simulink model "flat_earth_6dof"  (R2020b)
settings: Solver=FixedStepAuto  StartTime=0.0  StopTime=400  FixedStep=1/1000  MaxStep=0.01  RelTol=1e-5
model workspace (MATLAB code in the model file + MAT data in the model file):
  aeroCoeff.Cl0 = 0.000591
  aeroCoeff.Cl_beta = -0.0618
  aeroCoeff.Cl_da = -0.09917
  aeroCoeff.Cl_da_alpha = -0.08269
  aeroCoeff.Cl_dr = 0.006934
  aeroCoeff.Cl_p = -0.5045
  aeroCoeff.Cl_r = 0.1695
  aeroCoeff.Cm0 = 0.09448
  aeroCoeff.Cm_alpha = -0.6028
  aeroCoeff.Cm_alpha2 = -2.14
  aeroCoeff.Cm_beta2 = 0.6921
  aeroCoeff.Cm_de = -1.921
  aeroCoeff.Cm_df = 0.4072
  aeroCoeff.Cm_q = -15.56
  aeroCoeff.Cm_r = -0.3118
  aeroCoeff.Cn0 = -0.003117
  aeroCoeff.Cn_beta = 0.006719
  aeroCoeff.Cn_beta3 = 0.1373
  aeroCoeff.Cn_da = -0.003872
  aeroCoeff.Cn_dr = -0.08265
  aeroCoeff.Cn_p = -0.1585
  aeroCoeff.Cn_q = 0.1595
  aeroCoeff.Cn_r = -0.1112
  aeroCoeff.Cx0 = -0.03554
  aeroCoeff.Cx_alpha = 0.00292
  aeroCoeff.Cx_alpha2 = 5.459
  aeroCoeff.Cx_alpha3 = -5.162
  aeroCoeff.Cx_df = -0.09447
  aeroCoeff.Cx_df_alpha = 1.106
  aeroCoeff.Cx_dr = 0.03412
  aeroCoeff.Cx_q = -0.6748
  aeroCoeff.Cy0 = -0.002226
  aeroCoeff.Cy_beta = -0.7678
  aeroCoeff.Cy_da = -0.02956
  aeroCoeff.Cy_dr = 0.1158
  aeroCoeff.Cy_dr_alpha = 0.5238
  aeroCoeff.Cy_p = -0.124
  aeroCoeff.Cy_r = 0.3666
  aeroCoeff.Cz0 = -0.05504
  aeroCoeff.Cz_alpha = -5.578
  aeroCoeff.Cz_alpha3 = 3.442
  aeroCoeff.Cz_de = -0.398
  aeroCoeff.Cz_de_beta = -15.93
  aeroCoeff.Cz_df = -1.377
  aeroCoeff.Cz_df_alpha = -1.261
  aeroCoeff.Cz_q = -2.988
  environment.EarthRefAlt = 0
  initCond.x0 = [0 0 0]
  initCond.v0 = [0 0 0]
  initCond.euler0 = [0 0 0]
  initCond.w0 = [0 0 0]
  inputs0.time = 0
  inputs0.signals(1).dimensions = 1
  inputs0.signals(1).values = 0
  inputs0.signals(2).dimensions = 1
  inputs0.signals(2).values = 0
  inputs0.signals(3).dimensions = 1
  inputs0.signals(3).values = 0
  states0.time = 0
  states0.signals(1).values = [0 0 -2202]
  states0.signals(1).dimensions = 3
  states0.signals(1).label = 'CSTATE'
  states0.signals(1).blockName = 'asb6DOFAirframeTemplate/6DOF EOM/6DOF (Euler Angles)/xe,ye,ze'
  states0.signals(1).stateName = ''
  states0.signals(1).inReferencedModel = 0
  states0.signals(1).sampleTime = [0 0]
  states0.signals(2).values = [0.128665353089 0.259337659946 -0.178947917154]
  states0.signals(2).dimensions = 3
  states0.signals(2).label = 'CSTATE'
  states0.signals(2).blockName = 'asb6DOFAirframeTemplate/6DOF EOM/6DOF (Euler Angles)/Calculate DCM &
    | Euler Angles/phi
    | theta
    | psi'
  states0.signals(2).stateName = ''
  states0.signals(2).inReferencedModel = 0
  states0.signals(2).sampleTime = [0 0]
  states0.signals(3).values = [36.9119692666 8.10720863264 8.82591882596]
  states0.signals(3).dimensions = 3
  states0.signals(3).label = 'CSTATE'
  states0.signals(3).blockName = 'asb6DOFAirframeTemplate/6DOF EOM/6DOF (Euler Angles)/ub,vb,wb'
  states0.signals(3).stateName = ''
  states0.signals(3).inReferencedModel = 0
  states0.signals(3).sampleTime = [0 0]
  states0.signals(4).values = [0 0 0]
  states0.signals(4).dimensions = 3
  states0.signals(4).label = 'CSTATE'
  states0.signals(4).blockName = 'asb6DOFAirframeTemplate/6DOF EOM/6DOF (Euler Angles)/p,q,r '
  states0.signals(4).stateName = ''
  states0.signals(4).inReferencedModel = 0
  states0.signals(4).sampleTime = [0 0]
  states0.signals(5).values = [0 0]
  states0.signals(5).dimensions = 2
  states0.signals(5).label = 'CSTATE'
  states0.signals(5).blockName = 'asb6DOFAirframeTemplate/Environment Model/Dryden Wind Turbulence Model 
    | (Continuous (+q +r))/Filters on velocities/Hwgw(s)/wg_p1'
  states0.signals(5).stateName = ''
  states0.signals(5).inReferencedModel = 0
  states0.signals(5).sampleTime = [0 0]
  states0.signals(6).values = [0 0]
  states0.signals(6).dimensions = 2
  states0.signals(6).label = 'CSTATE'
  states0.signals(6).blockName = 'asb6DOFAirframeTemplate/Environment Model/Dryden Wind Turbulence Model 
    | (Continuous (+q +r))/Filters on velocities/Hwgw(s)/wg_p2'
  states0.signals(6).stateName = ''
  states0.signals(6).inReferencedModel = 0
  states0.signals(6).sampleTime = [0 0]
  states0.signals(7).values = [0 0]
  states0.signals(7).dimensions = 2
  states0.signals(7).label = 'CSTATE'
  states0.signals(7).blockName = 'asb6DOFAirframeTemplate/Environment Model/Dryden Wind Turbulence Model 
    | (Continuous (+q +r))/Filters on velocities/Hvgw(s)/vg_p1'
  states0.signals(7).stateName = ''
  states0.signals(7).inReferencedModel = 0
  states0.signals(7).sampleTime = [0 0]
  states0.signals(8).values = [0 0]
  states0.signals(8).dimensions = 2
  states0.signals(8).label = 'CSTATE'
  states0.signals(8).blockName = 'asb6DOFAirframeTemplate/Environment Model/Dryden Wind Turbulence Model 
    | (Continuous (+q +r))/Filters on velocities/Hvgw(s)/vgw_p2'
  states0.signals(8).stateName = ''
  states0.signals(8).inReferencedModel = 0
  states0.signals(8).sampleTime = [0 0]
  states0.signals(9).values = [0 0]
  states0.signals(9).dimensions = 2
  states0.signals(9).label = 'CSTATE'
  states0.signals(9).blockName = 'asb6DOFAirframeTemplate/Environment Model/Dryden Wind Turbulence Model 
    | (Continuous (+q +r))/Filters on velocities/Hugw(s)/ug_p'
  states0.signals(9).stateName = ''
  states0.signals(9).inReferencedModel = 0
  states0.signals(9).sampleTime = [0 0]
  states0.signals(10).values = [0 0]
  states0.signals(10).dimensions = 2
  states0.signals(10).label = 'CSTATE'
  states0.signals(10).blockName = 'asb6DOFAirframeTemplate/Environment Model/Dryden Wind Turbulence Model 
    | (Continuous (+q +r))/Filters on angular rates/Hrgw/rgw_p'
  states0.signals(10).stateName = ''
  states0.signals(10).inReferencedModel = 0
  states0.signals(10).sampleTime = [0 0]
  states0.signals(11).values = [0 0]
  states0.signals(11).dimensions = 2
  states0.signals(11).label = 'CSTATE'
  states0.signals(11).blockName = 'asb6DOFAirframeTemplate/Environment Model/Dryden Wind Turbulence Model 
    | (Continuous (+q +r))/Filters on angular rates/Hqgw/qgw_p'
  states0.signals(11).stateName = ''
  states0.signals(11).inReferencedModel = 0
  states0.signals(11).sampleTime = [0 0]
  states0.signals(12).values = [0 0]
  states0.signals(12).dimensions = 2
  states0.signals(12).label = 'CSTATE'
  states0.signals(12).blockName = 'asb6DOFAirframeTemplate/Environment Model/Dryden Wind Turbulence Model 
    | (Continuous (+q +r))/Filters on angular rates/Hpgw/pgw_p'
  states0.signals(12).stateName = ''
  states0.signals(12).inReferencedModel = 0
  states0.signals(12).sampleTime = [0 0]
  vehicle.Sref = 23.23
  vehicle.cbar = 1.5875
  vehicle.bref = 14.63
  vehicle.CG = [0 0 0]
  vehicle.CP = [0 0 0]
  vehicle.inertia = [1  0  0; 0  0.144  0; 0  0  1]
  vehicle.acMass = 0.909090909091
  vehicle.Thrust = 2300
  vehicle.aileron_max = 0.523598775598
  vehicle.aileron_min = -0.523598775598
  vehicle.elevator_max = 0.523598775598
  vehicle.elevator_min = -0.523598775598
  vehicle.rudder_max = 1.0471975512
  vehicle.rudder_min = -1.0471975512
  other statements: initialize6DOFSkyHogg;
undefined symbols (not defined in the file or in its folder): Altitude_t, cgf, cgi, dref, mdot, mf, mi, sref, tburn, Thrusts
libraries: aerolibasang x6, aerolibatmos2 x2, shared6dof x1, aerolibwind2 x1
settings Model: SimulationMode=accelerator  Creator=natha  LastModifiedBy=natha
settings SolverCC: AutoInsertRateTranBlk=on  InsertRTBMode=Never (minimum delay)  MinimalZcImpactIntegration=on
settings DataIOCC: ExternalInput=inputs0  InitialState=states0  SaveFormat=Array  SaveOutput=off  ReturnWorkspaceOutputs=off
settings OptimizationCC: EnhancedBackFolding=on  StrengthReduction=on  InitFltsAndDblsToZero=on  DifferentSizesBufferReuse=on
settings DebuggingCC: WriteAfterWriteMsg=DisableAll  AlgebraicLoopMsg=none  FcnCallInpInsideContextMsg=warning  UnconnectedInputMsg=none  UnconnectedOutputMsg=none  UnconnectedLineMsg=none  UniqueDataStoreMsg=error  RootOutportRequireBusObject=none  StateNameClashWarn=warning  StrictBusMsg=ErrorOnBusTreatedAsVector  SFUnexpectedBacktrackingDiag=warning  SFNoUnconditionalDefaultTransitionDiag=warning  SFExecutionAtInitializationDiag=none  ArithmeticOperatorsInVariantConditions=warning
settings ModelReferenceCC: PropagateSignalLabelsOutOfModel=off
settings SFSimCC: SimUseLocalCustomCode=off
settings RTWCC: RTWUseLocalCustomCode=off
settings CodeAppCC: StateflowObjectComments=on

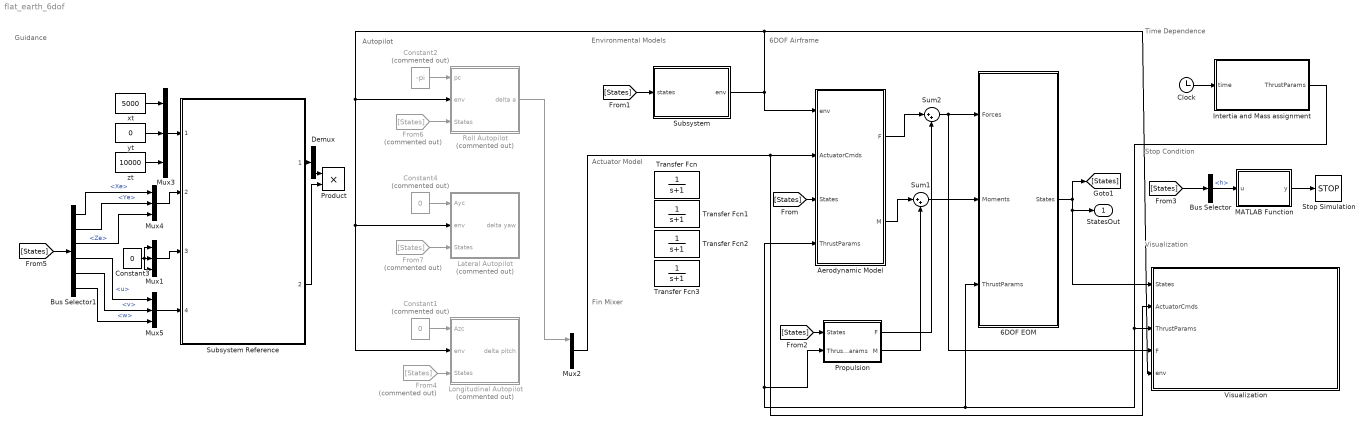
== system flat_earth_6dof ==
  note: 6DOF Airframe
  note: Environmental Models
  note: Autopilot
  note: Visualization
  note: Time Dependence
  note: Guidance
  note: Stop Condition
  note: Fin Mixer
  note: Actuator Model
  6DOF EOM : Subsystem  VariantControl=eom3DOF
  Aerodynamic Model : Subsystem  VariantControl=aeroCONST
  Bus Selector : BusSelector  OutputSignals=h
  Bus Selector1 : BusSelector  OutputSignals=Xe,Ye,Ze,u,v,w
  Clock : Clock
  Constant1 : Constant  Commented=on  Value=0
  Constant2 : Constant  Commented=on  Value=-pi
  Constant3 : Constant  Value=0
  Constant4 : Constant  Commented=on  Value=0
  Demux : Demux  Outputs=3
  From4 : From  Commented=on  GotoTag=States
  From6 : From  Commented=on  GotoTag=States
  From7 : From  Commented=on  GotoTag=States
  Intertia and Mass assignment : Subsystem
  Lateral Autopilot : Subsystem  Commented=on
  Longitudinal Autopilot : Subsystem  Commented=on
  MATLAB Function : MATLAB Function  TreatAsAtomicUnit=on
  Mux{1..5} (5 alike) : Mux  Inputs=3
  Product : Product
  Propulsion : Subsystem
      settings: RTWSystemCode=Inline
  Roll Autopilot : Subsystem  Commented=on
  Stop Simulation : Stop
  Subsystem : Subsystem
  Subsystem Reference : Subsystem  ReferencedSubsystem=PurePursuit
  Sum1 : Sum  Inputs=|++  InputSameDT=on  SaturateOnIntegerOverflow=on  OutDataTypeStr=Inherit: Same as first input
  Sum2 : Sum  Inputs=|++  InputSameDT=on  SaturateOnIntegerOverflow=on  OutDataTypeStr=Inherit: Same as first input
  Transfer Fcn{,1..3} (4 alike) : TransferFcn  Denominator=[1 1]
  Visualization : Subsystem
  xt : Constant  Value=5000
  yt : Constant  Value=0
  zt : Constant  Value=10000
  StatesOut : Outport  OutDataTypeStr=double  VectorParamsAs1DForOutWhenUnconnected=off
  wires:
  [States] -> Aerodynamic Model/3(States)
  Propulsion/2(M) -> Sum1/2
  [States] -> Propulsion/1(States)
  Intertia and Mass assignment/1(ThrustParams) -> 6DOF EOM/3(ThrustParams), Propulsion/2(ThrustParams), Aerodynamic Model/4(ThrustParams), Visualization/3(ThrustParams)
  Sum2/1 -> 6DOF EOM/1(Forces), Visualization/4(F)
  Aerodynamic Model/2(M) -> Sum1/1
  Propulsion/1(F) -> Sum2/2
  [States] -> Subsystem/1(states)
  Subsystem/1(env) -> Aerodynamic Model/1(env), Roll Autopilot/2(env), Lateral Autopilot/2(env), Longitudinal Autopilot/2(env), Visualization/5(env)
  MATLAB Function/1(y) -> Stop Simulation/1
  [States] -> Bus Selector/1
  Bus Selector/1 -> MATLAB Function/1(u)  "<h>"
  Clock/1 -> Intertia and Mass assignment/1(time)
  From4/1 -> Longitudinal Autopilot/3(States)
  Aerodynamic Model/1(F) -> Sum2/1
  Sum1/1 -> 6DOF EOM/2(Moments)
  Mux1/1 -> Subsystem Reference/3
  Constant3/1 -> Mux1/1, Mux1/2, Mux1/3
  Mux3/1 -> Subsystem Reference/1
  zt/1 -> Mux3/3
  yt/1 -> Mux3/2
  xt/1 -> Mux3/1
  [States] -> Bus Selector1/1
  Mux4/1 -> Subsystem Reference/2
  Bus Selector1/1 -> Mux4/1  "<Xe>"
  Bus Selector1/2 -> Mux4/2  "<Ye>"
  Bus Selector1/3 -> Mux4/3  "<Ze>"
  Mux5/1 -> Subsystem Reference/4
  Bus Selector1/4 -> Mux5/1  "<u>"
  Bus Selector1/5 -> Mux5/2  "<v>"
  Bus Selector1/6 -> Mux5/3  "<w>"
  Subsystem Reference/1 -> Demux/1
  Subsystem Reference/2 -> Product/2
  Demux/3 -> Product/1
  6DOF EOM/1(States) -> Visualization/1(States), StatesOut/1, [States]
  Constant1/1 -> Longitudinal Autopilot/1(Azc)
  Mux2/1 -> Aerodynamic Model/2(ActuatorCmds), Visualization/2(ActuatorCmds)
  From6/1 -> Roll Autopilot/3(States)
  From7/1 -> Lateral Autopilot/3(States)
  Constant4/1 -> Lateral Autopilot/1(Ayc)
  Constant2/1 -> Roll Autopilot/1(pc)
  Roll Autopilot/1(delta a) -> Mux2/1

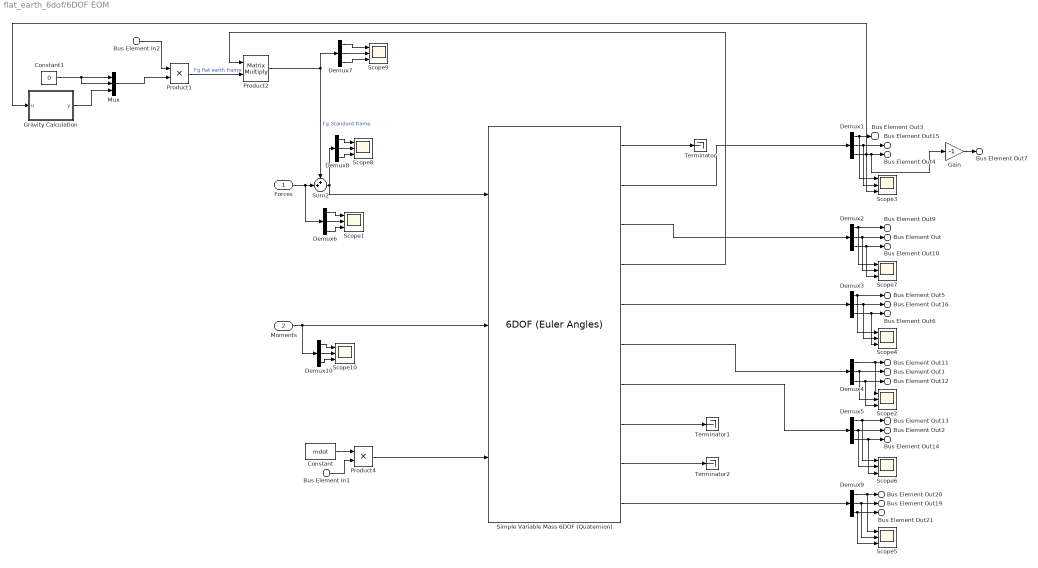
== system flat_earth_6dof/6DOF EOM ==
  Forces : Inport
  Moments : Inport  Port=2
  Bus Element In2 : Inport  Port=3  PortName=ThrustParams  Element=mass
  Bus Element In1 : Inport  Port=3  PortName=ThrustParams  Element=ThrustOn
  Constant : Constant  Value=mdot
  Constant1 : Constant  Value=0
  Demux{1..10} (10 alike) : Demux  Outputs=3
  Gain : Gain  Gain=-1
  Gravity Calculation : MATLAB Function  TreatAsAtomicUnit=on
  Mux : Mux  Inputs=3
  Product1 : Product
  Product2 : Product  Multiplication=Matrix(*)
  Product4 : Product
  Scope{1..10} (10 alike) : Scope  NumInputPorts=3
  Simple Variable Mass 6DOF (Quaternion) : shared6dof/6DOF (Euler Angles)  units=Metric (MKS)  mtype=Simple Variable  rep=Quaternion  xme_0=[0 0 -10000]  Vm_0=[0.0001 0 0]  eul_0=[0 45*(pi/180) 0]  pm_0=[0 0 0]  mass_0=mi  mass_e=mf  mass_f=mi  inertia=eye(3)  inertia_e=If  inertia_f=Ii  k_quat=1.0  vre_flag=off  abi_flag=on  aMode=0  xme_statename=''  Vm_statename=''  eul_statename=''  quat_statename=''  pm_statename=''  mass_statename=''
      settings: SourceProductBaseCode=AE,PW,MT,UV,VE,VP
  Sum2 : Sum  Inputs=++|  InputSameDT=on  SaturateOnIntegerOverflow=on  OutDataTypeStr=Inherit: Same as first input
  Terminator : Terminator
  Terminator1 : Terminator
  Terminator2 : Terminator
  Bus Element Out3 : Outport  VectorParamsAs1DForOutWhenUnconnected=off  PortName=States  Element=Xe
  Bus Element Out4 : Outport  VectorParamsAs1DForOutWhenUnconnected=off  PortName=States  Element=Ze
  Bus Element Out : Outport  VectorParamsAs1DForOutWhenUnconnected=off  PortName=States  Element=theta
  Bus Element Out5 : Outport  VectorParamsAs1DForOutWhenUnconnected=off  PortName=States  Element=u
  Bus Element Out6 : Outport  VectorParamsAs1DForOutWhenUnconnected=off  PortName=States  Element=w
  Bus Element Out1 : Outport  VectorParamsAs1DForOutWhenUnconnected=off  PortName=States  Element=q
  Bus Element Out2 : Outport  VectorParamsAs1DForOutWhenUnconnected=off  PortName=States  Element=q_dot
  Bus Element Out15 : Outport  VectorParamsAs1DForOutWhenUnconnected=off  PortName=States  Element=Ye
  Bus Element Out9 : Outport  VectorParamsAs1DForOutWhenUnconnected=off  PortName=States  Element=phi
  Bus Element Out10 : Outport  VectorParamsAs1DForOutWhenUnconnected=off  PortName=States  Element=psi
  Bus Element Out16 : Outport  VectorParamsAs1DForOutWhenUnconnected=off  PortName=States  Element=v
  Bus Element Out11 : Outport  VectorParamsAs1DForOutWhenUnconnected=off  PortName=States  Element=p
  Bus Element Out12 : Outport  VectorParamsAs1DForOutWhenUnconnected=off  PortName=States  Element=r
  Bus Element Out13 : Outport  VectorParamsAs1DForOutWhenUnconnected=off  PortName=States  Element=p_dot
  Bus Element Out14 : Outport  VectorParamsAs1DForOutWhenUnconnected=off  PortName=States  Element=r_dot
  Bus Element Out19 : Outport  VectorParamsAs1DForOutWhenUnconnected=off  PortName=States  Element=Ay
  Bus Element Out20 : Outport  VectorParamsAs1DForOutWhenUnconnected=off  PortName=States  Element=Ax
  Bus Element Out21 : Outport  VectorParamsAs1DForOutWhenUnconnected=off  PortName=States  Element=Az
  Bus Element Out7 : Outport  VectorParamsAs1DForOutWhenUnconnected=off  PortName=States  Element=h
  wires:
  Demux5/3 -> Scope6/3, Bus Element Out14/1
  Demux5/2 -> Bus Element Out2/1, Scope6/2
  Demux4/3 -> Scope2/3, Bus Element Out12/1
  Demux4/2 -> Bus Element Out1/1, Scope2/2
  Demux4/1 -> Scope2/1, Bus Element Out11/1
  Demux3/3 -> Scope4/3, Bus Element Out6/1
  Demux3/2 -> Scope4/2, Bus Element Out16/1
  Demux3/1 -> Scope4/1, Bus Element Out5/1
  Demux2/3 -> Scope7/3, Bus Element Out10/1
  Demux2/2 -> Scope7/2, Bus Element Out/1
  Demux2/1 -> Bus Element Out9/1, Scope7/1
  Demux1/3 -> Gravity Calculation/1(u), Scope3/3, Gain/1, Bus Element Out4/1
  Demux1/2 -> Scope3/2, Bus Element Out15/1
  Moments/1 -> Demux10/1, Simple Variable Mass 6DOF (Quaternion)/2
  Forces/1 -> Demux6/1, Sum2/2
  Bus Element In2/1 -> Product1/1
  Demux1/1 -> Scope3/1, Bus Element Out3/1
  Sum2/1 -> Simple Variable Mass 6DOF (Quaternion)/1, Demux8/1
  Demux9/2 -> Scope5/2, Bus Element Out19/1
  Demux9/3 -> Bus Element Out21/1, Scope5/3
  Demux9/1 -> Scope5/1, Bus Element Out20/1
  Demux5/1 -> Scope6/1, Bus Element Out13/1
  Demux6/1 -> Scope1/1
  Demux6/3 -> Scope1/3
  Demux6/2 -> Scope1/2
  Demux8/3 -> Scope8/3
  Demux8/2 -> Scope8/2
  Demux8/1 -> Scope8/1
  Demux10/1 -> Scope10/1
  Demux10/2 -> Scope10/2
  Demux10/3 -> Scope10/3
  Demux7/2 -> Scope9/2
  Demux7/3 -> Scope9/3
  Demux7/1 -> Scope9/1
  Product2/1 -> Demux7/1, Sum2/1  "Fg Standard frame"
  Bus Element In1/1 -> Product4/2
  Constant/1 -> Product4/1
  Product4/1 -> Simple Variable Mass 6DOF (Quaternion)/3
  Constant1/1 -> Mux/2, Mux/1
  Product1/1 -> Product2/2  "Fg flat earth frame"
  Mux/1 -> Product1/2
  Gravity Calculation/1(y) -> Mux/3
  Simple Variable Mass 6DOF (Quaternion)/1 -> Terminator/1
  Simple Variable Mass 6DOF (Quaternion)/2 -> Demux1/1
  Simple Variable Mass 6DOF (Quaternion)/3 -> Demux2/1
  Simple Variable Mass 6DOF (Quaternion)/4 -> Product2/1
  Simple Variable Mass 6DOF (Quaternion)/5 -> Demux3/1
  Simple Variable Mass 6DOF (Quaternion)/6 -> Demux4/1
  Simple Variable Mass 6DOF (Quaternion)/7 -> Demux5/1
  Simple Variable Mass 6DOF (Quaternion)/9 -> Terminator2/1
  Simple Variable Mass 6DOF (Quaternion)/8 -> Terminator1/1
  Simple Variable Mass 6DOF (Quaternion)/10 -> Demux9/1
  Gain/1 -> Bus Element Out7/1

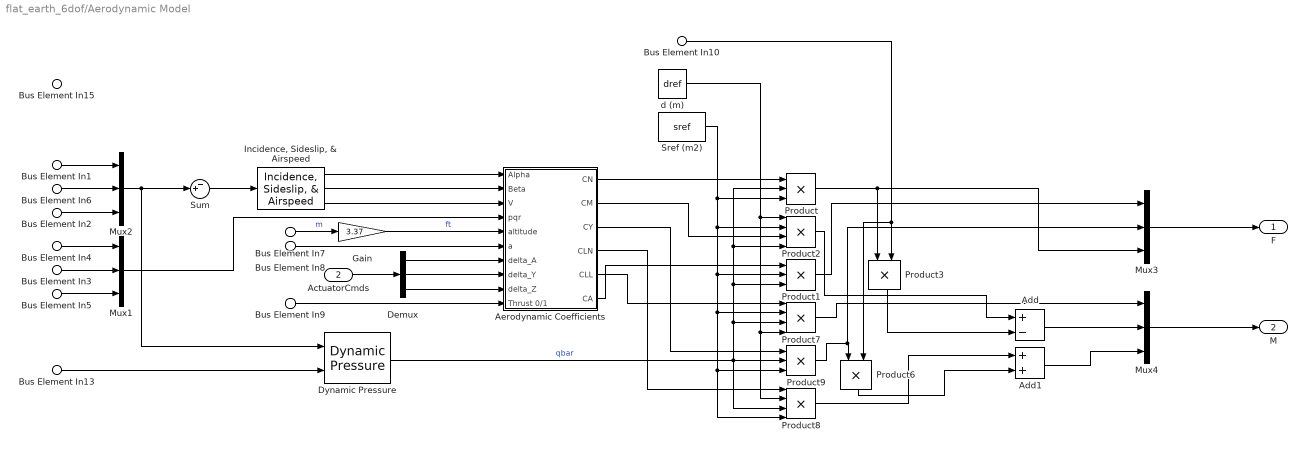
== system flat_earth_6dof/Aerodynamic Model ==
  Bus Element In13 : Inport  PortName=env  Element=rho
  Bus Element In8 : Inport  PortName=env  Element=a
  Bus Element In15 : Inport  PortName=env  Element=Vwind
  ActuatorCmds : Inport  Port=2
  Bus Element In1 : Inport  Port=3  PortName=States  Element=u
  Bus Element In2 : Inport  Port=3  PortName=States  Element=w
  Bus Element In3 : Inport  Port=3  PortName=States  Element=q
  Bus Element In6 : Inport  Port=3  PortName=States  Element=v
  Bus Element In4 : Inport  Port=3  PortName=States  Element=p
  Bus Element In5 : Inport  Port=3  PortName=States  Element=r
  Bus Element In7 : Inport  Port=3  PortName=States  Element=h
  Bus Element In9 : Inport  Port=4  PortName=ThrustParams  Element=ThrustOn
  Bus Element In10 : Inport  Port=4  PortName=ThrustParams  Element=cg
  Add : Sum  Inputs=+-
  Add1 : Sum
  Aerodynamic Coefficients : Subsystem
  Demux : Demux  Outputs=3
  Dynamic Pressure : aerolibasang/Dynamic Pressure
  Gain : Gain  Gain=3.37
  "Incidence, Sideslip, & Airspeed" : aerolibasang/Incidence, Sideslip, & Airspeed
  Mux{1..4} (4 alike) : Mux  Inputs=3
  Product : Product  Inputs=3
  Product1 : Product  Inputs=3
  Product2 : Product  Inputs=4
  Product3 : Product
  Product6 : Product
  Product7 : Product  Inputs=4
  Product8 : Product  Inputs=4
  Product9 : Product  Inputs=3
  Sref (m2) : Constant  Value=sref
  Sum : Sum  Inputs=-+|
  d (m) : Constant  Value=dref
  F : Outport  Unit=N  VectorParamsAs1DForOutWhenUnconnected=off
  M : Outport  Port=2  Unit=N*m  VectorParamsAs1DForOutWhenUnconnected=off
  wires:
  Bus Element In5/1 -> Mux1/3
  Bus Element In3/1 -> Mux1/2
  Bus Element In4/1 -> Mux1/1
  Mux1/1 -> Aerodynamic Coefficients/4(pqr)
  Mux2/1 -> Sum/2, Dynamic Pressure/1
  Dynamic Pressure/1 -> Product7/3, Product1/3, Product2/4, Product/2, Product8/3, Product9/2  "qbar"
  Bus Element In13/1 -> Dynamic Pressure/2
  "Incidence, Sideslip, & Airspeed"/3 -> Aerodynamic Coefficients/3(V)
  Bus Element In1/1 -> Mux2/1
  Bus Element In6/1 -> Mux2/2
  Bus Element In2/1 -> Mux2/3
  ActuatorCmds/1 -> Demux/1
  Demux/2 -> Aerodynamic Coefficients/8(delta_Y)
  Bus Element In8/1 -> Aerodynamic Coefficients/6(a)
  Sref (m2)/1 -> Product/3, Product8/4, Product9/3, Product7/2, Product1/2, Product2/2
  d (m)/1 -> Product8/2, Product7/4, Product2/1
  Product2/1 -> Add/1
  Product3/1 -> Add/2
  Bus Element In10/1 -> Product6/2, Product3/2
  Product1/1 -> Mux3/1
  Bus Element In7/1 -> Gain/1  "m"
  "Incidence, Sideslip, & Airspeed"/1 -> Aerodynamic Coefficients/1(Alpha)
  Product/1 -> Mux3/3, Product3/1
  Mux3/1 -> F/1
  Mux4/1 -> M/1
  "Incidence, Sideslip, & Airspeed"/2 -> Aerodynamic Coefficients/2(Beta)
  Aerodynamic Coefficients/1(CN) -> Product/1
  Aerodynamic Coefficients/2(CM) -> Product2/3
  Aerodynamic Coefficients/6(CA) -> Product1/1
  Product6/1 -> Add1/2
  Aerodynamic Coefficients/5(CLL) -> Product7/1
  Product7/1 -> Mux4/1
  Add1/1 -> Mux4/3
  Product9/1 -> Mux3/2, Product6/1
  Add/1 -> Mux4/2
  Product8/1 -> Add1/1
  Demux/3 -> Aerodynamic Coefficients/9(delta_Z)
  Gain/1 -> Aerodynamic Coefficients/5(altitude)  "ft"
  Sum/1 -> "Incidence, Sideslip, & Airspeed"/1
  Bus Element In9/1 -> Aerodynamic Coefficients/10(Thrust 0/1)
  Demux/1 -> Aerodynamic Coefficients/7(delta_A)
  Aerodynamic Coefficients/4(CLN) -> Product8/1
  Aerodynamic Coefficients/3(CY) -> Product9/1

== system flat_earth_6dof/Intertia and Mass assignment ==
  time : Inport
  Constant : Constant  Value=tburn
  Constant1 : Constant  Value=mi
  Constant2 : Constant  Value=mf
  Constant3 : Constant  Value=mdot
  Constant4 : Constant  Value=cgi
  Constant5 : Constant  Value=cgf
  MATLAB Function1 : MATLAB Function  TreatAsAtomicUnit=on
  MATLAB Function2 : MATLAB Function  TreatAsAtomicUnit=on
  MATLAB Function3 : MATLAB Function  TreatAsAtomicUnit=on
  Mux : Mux  Inputs=7
  Out Bus Element : Outport  PortName=ThrustParams  Element=ThrustOn
  Out Bus Element1 : Outport  PortName=ThrustParams  Element=mass
  Out Bus Element2 : Outport  PortName=ThrustParams  Element=cg
  wires:
  MATLAB Function2/1(y) -> Out Bus Element/1
  MATLAB Function1/1(y) -> Out Bus Element1/1
  MATLAB Function3/1(y) -> Out Bus Element2/1
  Constant2/1 -> Mux/4
  Constant1/1 -> Mux/3
  Constant/1 -> Mux/2
  time/1 -> Mux/1
  Constant3/1 -> Mux/5
  Constant4/1 -> Mux/6
  Constant5/1 -> Mux/7
  Mux/1 -> MATLAB Function3/1(u), MATLAB Function2/1(u), MATLAB Function1/1(u)

== system flat_earth_6dof/Lateral Autopilot ==
  Ayc : Inport
  env : Inport  Port=2
  States : Inport  Port=3
  3 loop autopilot : Subsystem
  Gain Scheduler : Subsystem
  delta yaw : Outport
  wires:
  Gain Scheduler/4(kss) -> 3 loop autopilot/6(kss)
  3 loop autopilot/1(delta yaw) -> delta yaw/1
  env/1 -> Gain Scheduler/1(env)
  Ayc/1 -> 3 loop autopilot/2(Ayc)
  Gain Scheduler/1(k1) -> 3 loop autopilot/3(k1)
  Gain Scheduler/3(k3) -> 3 loop autopilot/5(k3)
  Gain Scheduler/2(k2) -> 3 loop autopilot/4(k2)
  States/1 -> Gain Scheduler/2(States), 3 loop autopilot/1(States)

== system flat_earth_6dof/Longitudinal Autopilot ==
  Azc : Inport
  env : Inport  Port=2
  States : Inport  Port=3
  3 loop autopilot : Subsystem
  Gain Scheduler : Subsystem
  Scope : Scope
  delta pitch : Outport
  wires:
  Gain Scheduler/4(kss) -> 3 loop autopilot/6(kss)
  3 loop autopilot/1(deltap) -> Scope/1, delta pitch/1  "Pitch"
  env/1 -> Gain Scheduler/1(env)
  States/1 -> Gain Scheduler/2(States), 3 loop autopilot/1(States)
  Azc/1 -> 3 loop autopilot/2(Azc)
  Gain Scheduler/1(k1) -> 3 loop autopilot/3(k1)
  Gain Scheduler/3(k3) -> 3 loop autopilot/5(k3)
  Gain Scheduler/2(k2) -> 3 loop autopilot/4(k2)

== system flat_earth_6dof/Propulsion ==
  Bus Element In : Inport  PortName=States  Element=h
  Bus Element In2 : Inport  Port=2  PortName=ThrustParams  Element=ThrustOn
  Constant : Constant  Value=0
  Constant1 : Constant  Value=0
  Mux : Mux  Inputs=3
  Product : Product
  ThrustX : Lookup_n-D  NumberOfTableDimensions=1  LookupTableObject=''  BreakpointsForDimension1=Altitude_t  IndexSearchMethod=Linear search  BeginIndexSearchUsingPreviousIndexResult=on  Table=Thrusts  ExtrapMethod=Clip  UseLastTableValue=on  InputSameDT=on
  Thrust_M1 : Constant  Value=[0 0 0]'  SampleTime=-1
  F : Outport  Unit=N  VectorParamsAs1DForOutWhenUnconnected=off
  M : Outport  Port=2  Unit=N*m  VectorParamsAs1DForOutWhenUnconnected=off
  wires:
  Thrust_M1/1 -> M/1
  Mux/1 -> F/1
  ThrustX/1 -> Product/1
  Bus Element In2/1 -> Product/2
  Product/1 -> Mux/1
  Constant1/1 -> Mux/3
  Constant/1 -> Mux/2
  Bus Element In/1 -> ThrustX/1

== system flat_earth_6dof/Roll Autopilot ==
  pc : Inport
  env : Inport  Port=2
  States : Inport  Port=3
  Gain Scheduler : Subsystem
  Roll autopilot : Subsystem
  delta a : Outport
  wires:
  Roll autopilot/1(delta a) -> delta a/1  "delta a"
  env/1 -> Gain Scheduler/1(env)
  States/1 -> Roll autopilot/1(States), Gain Scheduler/2(States)
  pc/1 -> Roll autopilot/2(pc)
  Gain Scheduler/1(k1) -> Roll autopilot/3(k1)
  Gain Scheduler/2(k2) -> Roll autopilot/4(k2)
  Gain Scheduler/3(kss) -> Roll autopilot/5(kss)

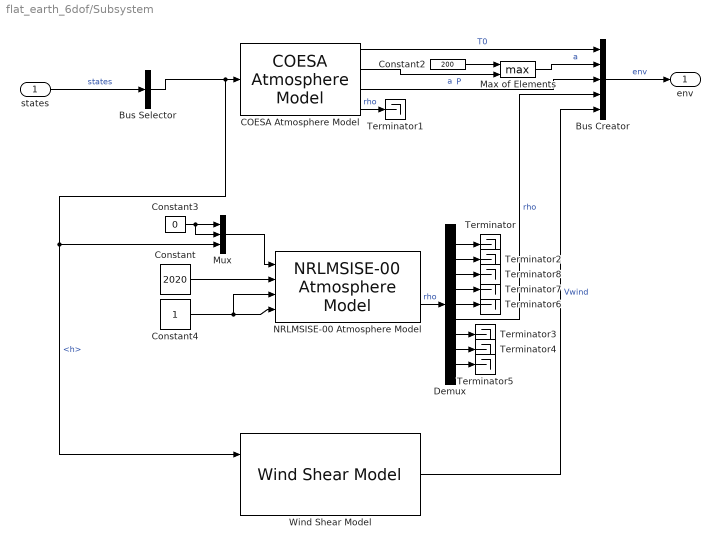
== system flat_earth_6dof/Subsystem ==
  states : Inport
  Bus Creator : BusCreator  Inputs=5
  Bus Selector : BusSelector  OutputSignals=h
  COESA Atmosphere Model : aerolibatmos2/COESA Atmosphere Model  units=Metric (MKS)  spec=1976 COESA-extended U.S. Standard Atmosphere  model=Profile  profile_var=High temperature  profile_percent=1%  profile_alt=5 km (16404 ft)  envelope_var=High temperature  envelope_percent=1%  action=Warning
  Constant : Constant  Value=2020
  Constant2 : Constant  Value=200
  Constant3 : Constant  Value=0
  Constant4 : Constant
  Demux : Demux  Outputs=9
  Max of Elements : MinMax  Function=max  Inputs=2
  Mux : Mux  Inputs=3
  NRLMSISE-00 Atmosphere Model : aerolibatmos2/NRLMSISE-00 Atmosphere Model  units=Metric (MKS)  lst_input=off  flux_ap_input=off  flags_input=Internal  flags=ones(1,23)  oxygen_in=off  action=Warning
      settings: SourceProductBaseCode=AE
  Terminator{,1..8} (9 alike) : Terminator
  Wind Shear Model : aerolibwind2/Wind Shear Model  units=Metric (MKS)  phase=Category C - Terminal Flight Phase  W_20=15  Wdeg=0
  env : Outport
  wires:
  states/1 -> Bus Selector/1  "states"
  COESA Atmosphere Model/3 -> Bus Creator/3  "P"
  COESA Atmosphere Model/2 -> Max of Elements/2  "a"
  Bus Selector/1 -> COESA Atmosphere Model/1, Mux/3, Wind Shear Model/1  "<h>"
  Bus Creator/1 -> env/1  "env"
  COESA Atmosphere Model/1 -> Bus Creator/1  "T0"
  Max of Elements/1 -> Bus Creator/2  "a"
  Constant2/1 -> Max of Elements/1
  Mux/1 -> NRLMSISE-00 Atmosphere Model/1
  Constant3/1 -> Mux/2, Mux/1
  Constant/1 -> NRLMSISE-00 Atmosphere Model/2
  Constant4/1 -> NRLMSISE-00 Atmosphere Model/3, NRLMSISE-00 Atmosphere Model/4
  NRLMSISE-00 Atmosphere Model/2 -> Demux/1  "rho"
  Demux/6 -> Bus Creator/4  "rho"
  Demux/1 -> Terminator/1
  COESA Atmosphere Model/4 -> Terminator1/1  "rho"
  Demux/2 -> Terminator2/1
  Demux/3 -> Terminator8/1
  Demux/4 -> Terminator7/1
  Demux/5 -> Terminator6/1
  Demux/7 -> Terminator3/1
  Demux/8 -> Terminator4/1
  Demux/9 -> Terminator5/1
  Wind Shear Model/1 -> Bus Creator/5  "Vwind"

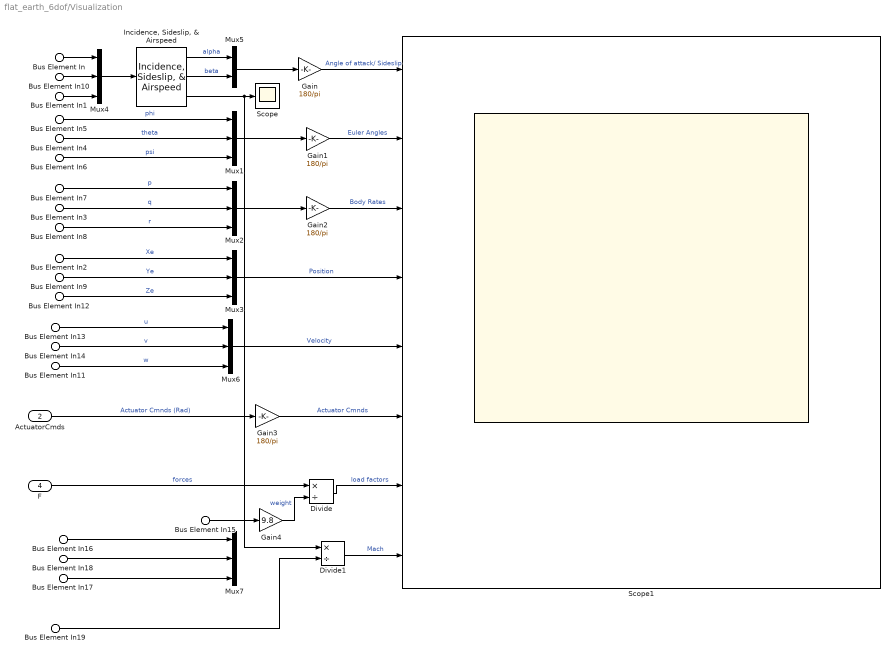
== system flat_earth_6dof/Visualization ==
  Bus Element In : Inport  PortName=States  Element=u
  Bus Element In13 : Inport  PortName=States  Element=u
  Bus Element In1 : Inport  PortName=States  Element=w
  Bus Element In11 : Inport  PortName=States  Element=w
  Bus Element In3 : Inport  PortName=States  Element=q
  Bus Element In4 : Inport  PortName=States  Element=theta
  Bus Element In12 : Inport  PortName=States  Element=Ze
  Bus Element In2 : Inport  PortName=States  Element=Xe
  Bus Element In10 : Inport  PortName=States  Element=v
  Bus Element In14 : Inport  PortName=States  Element=v
  Bus Element In5 : Inport  PortName=States  Element=phi
  Bus Element In6 : Inport  PortName=States  Element=psi
  Bus Element In7 : Inport  PortName=States  Element=p
  Bus Element In8 : Inport  PortName=States  Element=r
  Bus Element In9 : Inport  PortName=States  Element=Ye
  Bus Element In16 : Inport  PortName=States  Element=Ax
  Bus Element In18 : Inport  PortName=States  Element=Ay
  Bus Element In17 : Inport  PortName=States  Element=Az
  ActuatorCmds : Inport  Port=2
  Bus Element In15 : Inport  Port=3  PortName=ThrustParams  Element=mass
  F : Inport  Port=4
  Bus Element In19 : Inport  Port=5  PortName=env  Element=a
  Divide : Product  Inputs=*/
  Divide1 : Product  Inputs=*/
  Gain{,1..3} (4 alike) : Gain  Gain=180/pi
  Gain4 : Gain  Gain=9.8
  "Incidence, Sideslip, & Airspeed" : aerolibasang/Incidence, Sideslip, & Airspeed
  Mux{1..4,6..7} (6 alike) : Mux  Inputs=3
  Mux5 : Mux  Inputs=2
  Scope : Scope
  Scope1 : Scope  NumInputPorts=8
  wires:
  Mux3/1 -> Scope1/4  "Position"
  Bus Element In2/1 -> Mux3/1  "Xe"
  Bus Element In9/1 -> Mux3/2  "Ye"
  Bus Element In12/1 -> Mux3/3  "Ze"
  Mux2/1 -> Gain2/1
  Mux1/1 -> Gain1/1
  Mux5/1 -> Gain/1
  "Incidence, Sideslip, & Airspeed"/2 -> Mux5/2  "beta"
  "Incidence, Sideslip, & Airspeed"/1 -> Mux5/1  "alpha"
  Mux4/1 -> "Incidence, Sideslip, & Airspeed"/1
  Bus Element In10/1 -> Mux4/2
  Bus Element In8/1 -> Mux2/3  "r"
  Bus Element In7/1 -> Mux2/1  "p"
  Bus Element In6/1 -> Mux1/3  "psi"
  Bus Element In5/1 -> Mux1/1  "phi"
  Bus Element In4/1 -> Mux1/2  "theta"
  Bus Element In3/1 -> Mux2/2  "q"
  Bus Element In1/1 -> Mux4/3
  Bus Element In/1 -> Mux4/1
  "Incidence, Sideslip, & Airspeed"/3 -> Divide1/1, Scope/1
  Gain/1 -> Scope1/1  "Angle of attack/ Sideslip"
  Gain1/1 -> Scope1/2  "Euler Angles"
  Gain2/1 -> Scope1/3  "Body Rates"
  Mux6/1 -> Scope1/5  "Velocity"
  Bus Element In13/1 -> Mux6/1  "u"
  Bus Element In14/1 -> Mux6/2  "v"
  Bus Element In11/1 -> Mux6/3  "w"
  ActuatorCmds/1 -> Gain3/1  "Actuator Cmnds (Rad)"
  Gain3/1 -> Scope1/6  "Actuator Cmnds"
  Bus Element In17/1 -> Mux7/3
  Bus Element In18/1 -> Mux7/2
  Bus Element In16/1 -> Mux7/1
  F/1 -> Divide/1  "forces"
  Bus Element In15/1 -> Gain4/1
  Gain4/1 -> Divide/2  "weight"
  Divide/1 -> Scope1/7  "load factors"
  Bus Element In19/1 -> Divide1/2
  Divide1/1 -> Scope1/8  "Mach"

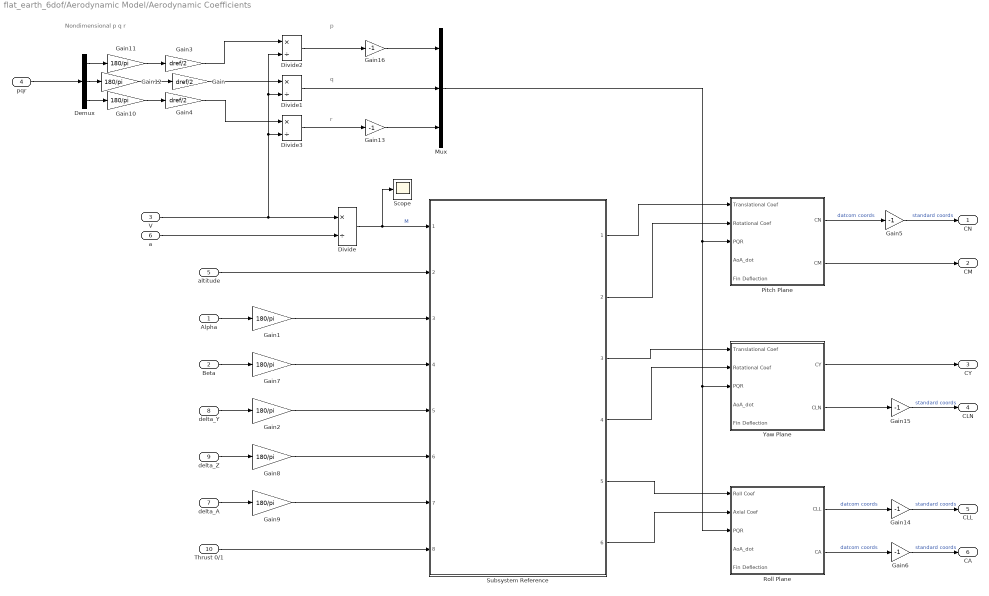
== system flat_earth_6dof/Aerodynamic Model/Aerodynamic Coefficients ==
  note: q
  note: p
  note: Nondimensional p q r
  note: r
  Alpha : Inport
  Beta : Inport  Port=2
  V : Inport  Port=3
  pqr : Inport  Port=4  Unit=1/s
  altitude : Inport  Port=5
  a : Inport  Port=6
  delta_A : Inport  Port=7
  delta_Y : Inport  Port=8
  delta_Z : Inport  Port=9
  Thrust 0/1 : Inport  Port=10
  Demux : Demux  Outputs=3
  Divide{,1..3} (4 alike) : Product  Inputs=*/
  Gain : Gain  Gain=dref/2
  Gain{1..2,7..12} (8 alike) : Gain  Gain=180/pi
  Gain{5..6,13..16} (6 alike) : Gain  Gain=-1
  Gain3 : Gain  Gain=dref/2
  Gain4 : Gain  Gain=dref/2
  Mux : Mux  Inputs=3
  Pitch Plane : Subsystem
  Roll Plane : Subsystem
  Scope : Scope
  Subsystem Reference : Subsystem  ReferencedSubsystem=AeroCoefficientsFull
  Yaw Plane : Subsystem
  CN : Outport  VectorParamsAs1DForOutWhenUnconnected=off
  CM : Outport  Port=2  VectorParamsAs1DForOutWhenUnconnected=off
  CY : Outport  Port=3  VectorParamsAs1DForOutWhenUnconnected=off
  CLN : Outport  Port=4  VectorParamsAs1DForOutWhenUnconnected=off
  CLL : Outport  Port=5  VectorParamsAs1DForOutWhenUnconnected=off
  CA : Outport  Port=6  VectorParamsAs1DForOutWhenUnconnected=off
  wires:
  a/1 -> Divide/2
  V/1 -> Divide1/2, Divide2/2, Divide3/2, Divide/1
  Divide/1 -> Scope/1, Subsystem Reference/1  "M"
  altitude/1 -> Subsystem Reference/2
  pqr/1 -> Demux/1
  Alpha/1 -> Gain1/1
  Gain1/1 -> Subsystem Reference/3
  delta_Y/1 -> Gain2/1
  Gain/1 -> Divide1/1
  Gain2/1 -> Subsystem Reference/5
  delta_Z/1 -> Gain8/1
  delta_A/1 -> Gain9/1
  Thrust 0/1/1 -> Subsystem Reference/8
  Demux/3 -> Gain10/1
  Demux/1 -> Gain11/1
  Gain3/1 -> Divide2/1
  Gain4/1 -> Divide3/1
  Divide1/1 -> Mux/2
  Divide3/1 -> Gain13/1
  Subsystem Reference/1 -> Pitch Plane/1(Translational Coef)
  Subsystem Reference/2 -> Pitch Plane/2(Rotational Coef)
  Subsystem Reference/3 -> Yaw Plane/1(Translational Coef)
  Subsystem Reference/4 -> Yaw Plane/2(Rotational Coef)
  Subsystem Reference/6 -> Roll Plane/2(Axial Coef)
  Yaw Plane/1(CY) -> CY/1
  Mux/1 -> Roll Plane/3(PQR), Yaw Plane/3(PQR), Pitch Plane/3(PQR)
  Subsystem Reference/5 -> Roll Plane/1(Roll Coef)
  Roll Plane/2(CA) -> Gain6/1  "datcom coords"
  Gain6/1 -> CA/1  "standard coords"
  Pitch Plane/1(CN) -> Gain5/1  "datcom coords"
  Gain5/1 -> CN/1  "standard coords"
  Gain7/1 -> Subsystem Reference/4
  Gain8/1 -> Subsystem Reference/6
  Gain10/1 -> Gain4/1
  Demux/2 -> Gain12/1
  Gain11/1 -> Gain3/1
  Gain12/1 -> Gain/1
  Yaw Plane/2(CLN) -> Gain15/1
  Beta/1 -> Gain7/1
  Pitch Plane/2(CM) -> CM/1
  Gain15/1 -> CLN/1  "standard coords"
  Gain13/1 -> Mux/3
  Roll Plane/1(CLL) -> Gain14/1  "datcom coords"
  Divide2/1 -> Gain16/1
  Gain14/1 -> CLL/1  "standard coords"
  Gain16/1 -> Mux/1
  Gain9/1 -> Subsystem Reference/7

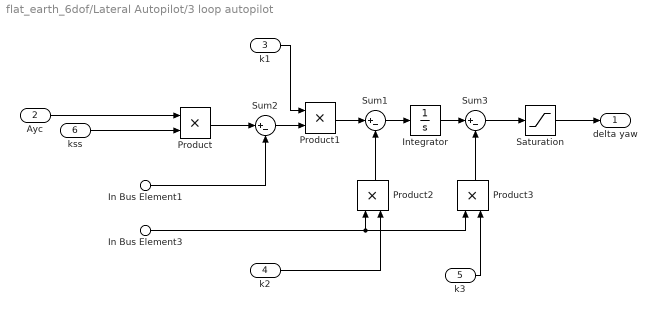
== system flat_earth_6dof/Lateral Autopilot/3 loop autopilot ==
  In Bus Element3 : Inport  PortName=States  Element=r
  In Bus Element1 : Inport  PortName=States  Element=Ay
  Ayc : Inport  Port=2
  k1 : Inport  Port=3
  k2 : Inport  Port=4
  k3 : Inport  Port=5
  kss : Inport  Port=6
  Integrator : Integrator
  Product{,1..3} (4 alike) : Product
  Saturation : Saturate  UpperLimit=15*(pi/90)  LowerLimit=-15*(pi/90)
  Sum1 : Sum  Inputs=|+-
  Sum2 : Sum  Inputs=|+-
  Sum3 : Sum  Inputs=|+-
  delta yaw : Outport
  wires:
  Ayc/1 -> Product/1
  k2/1 -> Product2/2
  In Bus Element3/1 -> Product3/1, Product2/1
  Product2/1 -> Sum1/2
  Sum3/1 -> Saturation/1
  Product/1 -> Sum2/1
  In Bus Element1/1 -> Sum2/2
  Sum2/1 -> Product1/2
  k1/1 -> Product1/1
  Sum1/1 -> Integrator/1
  Product1/1 -> Sum1/1
  Integrator/1 -> Sum3/1
  Product3/1 -> Sum3/2
  k3/1 -> Product3/2
  Saturation/1 -> delta yaw/1
  kss/1 -> Product/2

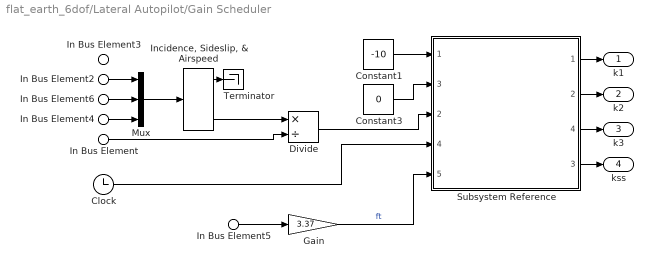
== system flat_earth_6dof/Lateral Autopilot/Gain Scheduler ==
  In Bus Element : Inport  PortName=env  Element=a
  In Bus Element2 : Inport  Port=2  PortName=States  Element=u
  In Bus Element6 : Inport  Port=2  PortName=States  Element=v
  In Bus Element4 : Inport  Port=2  PortName=States  Element=w
  In Bus Element5 : Inport  Port=2  PortName=States  Element=h
  In Bus Element3 : Inport  Port=2  PortName=States  Element=Ax
  Clock : Clock
  Constant1 : Constant  Value=-10
  Constant3 : Constant  Value=0
  Divide : Product  Inputs=*/
  Gain : Gain  Gain=3.37
  "Incidence, Sideslip, & Airspeed" : aerolibasang/Incidence, Sideslip, & Airspeed
  Mux : Mux  Inputs=3
  Subsystem Reference : Subsystem  ReferencedSubsystem=autopilot_subsys
      settings: PortSchema="{\"entries\":[{\"content\":{\"sides\":[{\"content\":{\"connectorIds\":[\"In1\",\"In3\",\"In2\",\"In4\",\"In5\"]},\"type\":\"ConnectorPlacement.EquallySpacedRectSide\",\"uuid\":\"480b0030-5dbb-4bdb-b5e0-81b840be2b57\"},{\"content\":{\"connectorIds\":[\"Out1\",\"Out2\",\"Out4\",\"Out3\"],\"side\":\"RIGHT\"},\"type\":\"ConnectorPlacement.EquallySpacedRectSide\",\"uuid\":\"1f12df62-2a0c-474c-bbce-f3fb9e29b135\"},{\"content\":{\"connectorIds\":[],\"side\":\"TOP\"},\"type\":\"ConnectorPlacement.EquallySpacedRectSide\",\"uuid\":\"a52c0cb6-b4f1-4ba5-8b18-9cab9a578b93\"},{\"content\":{\"connectorIds\":[],\"side\":\"HIDDEN\"},\"type\":\"ConnectorPlacement.EquallySpacedRectSide\",\"uuid\":\"3b18b842-e4ca-48ac-a811-1dbcab558bc6\"}]},\"type\":\"ConnectorPlacement.EquallySpacedConnector\",\"uuid\":\"1b930547-9173-4587-885f-ee6643b32fc8\"}],\"packageUris\":[\"http://schema.mathworks.com/mf0/Connector/R2020b\"],\"version\":\"1.0\"}"
  Terminator : Terminator
  k1 : Outport
  k2 : Outport  Port=2
  k3 : Outport  Port=3
  kss : Outport  Port=4
  wires:
  Subsystem Reference/1 -> k1/1
  Subsystem Reference/2 -> k2/1
  In Bus Element2/1 -> Mux/1
  In Bus Element6/1 -> Mux/2
  In Bus Element4/1 -> Mux/3
  Mux/1 -> "Incidence, Sideslip, & Airspeed"/1
  "Incidence, Sideslip, & Airspeed"/3 -> Divide/1
  In Bus Element/1 -> Divide/2
  Subsystem Reference/3 -> kss/1
  In Bus Element5/1 -> Gain/1
  Subsystem Reference/4 -> k3/1
  "Incidence, Sideslip, & Airspeed"/1 -> Terminator/1
  Divide/1 -> Subsystem Reference/2
  Constant1/1 -> Subsystem Reference/1
  Constant3/1 -> Subsystem Reference/3
  Clock/1 -> Subsystem Reference/4
  Gain/1 -> Subsystem Reference/5  "ft"

== system flat_earth_6dof/Longitudinal Autopilot/3 loop autopilot ==
  In Bus Element3 : Inport  PortName=States  Element=q
  In Bus Element1 : Inport  PortName=States  Element=Az
  Azc : Inport  Port=2
  k1 : Inport  Port=3
  k2 : Inport  Port=4
  k3 : Inport  Port=5
  kss : Inport  Port=6
  Integrator : Integrator
  Product{,1..3} (4 alike) : Product
  Saturation : Saturate  UpperLimit=15*(pi/90)  LowerLimit=-15*(pi/90)
  Sum1 : Sum  Inputs=|+-
  Sum2 : Sum  Inputs=|+-
  Sum3 : Sum  Inputs=|+-
  deltap : Outport
  wires:
  Azc/1 -> Product/1
  k2/1 -> Product2/2
  In Bus Element3/1 -> Product3/1, Product2/1
  Product2/1 -> Sum1/2
  Sum3/1 -> Saturation/1
  Product/1 -> Sum2/1
  In Bus Element1/1 -> Sum2/2
  Sum2/1 -> Product1/2
  k1/1 -> Product1/1
  Sum1/1 -> Integrator/1
  Product1/1 -> Sum1/1
  Integrator/1 -> Sum3/1
  Product3/1 -> Sum3/2
  k3/1 -> Product3/2
  Saturation/1 -> deltap/1
  kss/1 -> Product/2

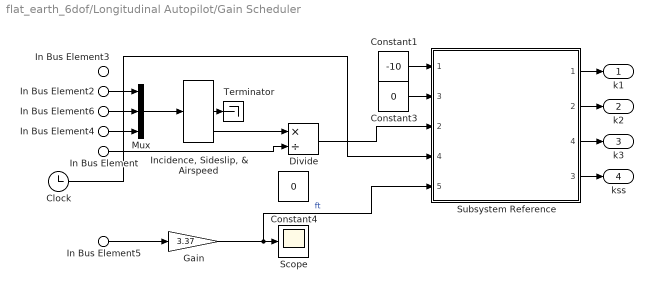
== system flat_earth_6dof/Longitudinal Autopilot/Gain Scheduler ==
  In Bus Element : Inport  PortName=env  Element=a
  In Bus Element2 : Inport  Port=2  PortName=States  Element=u
  In Bus Element6 : Inport  Port=2  PortName=States  Element=v
  In Bus Element4 : Inport  Port=2  PortName=States  Element=w
  In Bus Element5 : Inport  Port=2  PortName=States  Element=h
  In Bus Element3 : Inport  Port=2  PortName=States  Element=Ax
  Clock : Clock
  Constant1 : Constant  Value=-10
  Constant3 : Constant  Value=0
  Constant4 : Constant  Value=0
  Divide : Product  Inputs=*/
  Gain : Gain  Gain=3.37
  "Incidence, Sideslip, & Airspeed" : aerolibasang/Incidence, Sideslip, & Airspeed
  Mux : Mux  Inputs=3
  Scope : Scope
  Subsystem Reference : Subsystem  ReferencedSubsystem=autopilot_subsys
      settings: PortSchema="{\"entries\":[{\"content\":{\"sides\":[{\"content\":{\"connectorIds\":[\"In1\",\"In3\",\"In2\",\"In4\",\"In5\"]},\"type\":\"ConnectorPlacement.EquallySpacedRectSide\",\"uuid\":\"480b0030-5dbb-4bdb-b5e0-81b840be2b57\"},{\"content\":{\"connectorIds\":[\"Out1\",\"Out2\",\"Out4\",\"Out3\"],\"side\":\"RIGHT\"},\"type\":\"ConnectorPlacement.EquallySpacedRectSide\",\"uuid\":\"1f12df62-2a0c-474c-bbce-f3fb9e29b135\"},{\"content\":{\"connectorIds\":[],\"side\":\"TOP\"},\"type\":\"ConnectorPlacement.EquallySpacedRectSide\",\"uuid\":\"a52c0cb6-b4f1-4ba5-8b18-9cab9a578b93\"},{\"content\":{\"connectorIds\":[],\"side\":\"HIDDEN\"},\"type\":\"ConnectorPlacement.EquallySpacedRectSide\",\"uuid\":\"3b18b842-e4ca-48ac-a811-1dbcab558bc6\"}]},\"type\":\"ConnectorPlacement.EquallySpacedConnector\",\"uuid\":\"1b930547-9173-4587-885f-ee6643b32fc8\"}],\"packageUris\":[\"http://schema.mathworks.com/mf0/Connector/R2020b\"],\"version\":\"1.0\"}"
  Terminator : Terminator
  k1 : Outport
  k2 : Outport  Port=2
  k3 : Outport  Port=3
  kss : Outport  Port=4
  wires:
  Subsystem Reference/1 -> k1/1
  Subsystem Reference/2 -> k2/1
  In Bus Element2/1 -> Mux/1
  In Bus Element6/1 -> Mux/2
  In Bus Element4/1 -> Mux/3
  Mux/1 -> "Incidence, Sideslip, & Airspeed"/1
  "Incidence, Sideslip, & Airspeed"/3 -> Divide/1
  In Bus Element/1 -> Divide/2
  Divide/1 -> Subsystem Reference/2
  "Incidence, Sideslip, & Airspeed"/2 -> Terminator/1
  Subsystem Reference/3 -> kss/1
  Subsystem Reference/4 -> k3/1
  In Bus Element5/1 -> Gain/1
  Gain/1 -> Subsystem Reference/5, Scope/1  "ft"
  Clock/1 -> Subsystem Reference/4
  Constant1/1 -> Subsystem Reference/1
  Constant3/1 -> Subsystem Reference/3

== system flat_earth_6dof/Roll Autopilot/Gain Scheduler ==
  In Bus Element : Inport  PortName=env  Element=a
  In Bus Element2 : Inport  Port=2  PortName=States  Element=u
  In Bus Element6 : Inport  Port=2  PortName=States  Element=v
  In Bus Element4 : Inport  Port=2  PortName=States  Element=w
  In Bus Element5 : Inport  Port=2  PortName=States  Element=h
  Clock : Clock
  Constant1 : Constant  Value=0
  Divide : Product  Inputs=*/
  "Incidence, Sideslip, & Airspeed" : aerolibasang/Incidence, Sideslip, & Airspeed
  Mux : Mux  Inputs=3
  Subsystem Reference : Subsystem  ReferencedSubsystem=roll_autopilot_gain_scheduler
  Terminator : Terminator
  k1 : Outport
  k2 : Outport  Port=2
  kss : Outport  Port=3
  wires:
  Subsystem Reference/1 -> k1/1
  Subsystem Reference/2 -> k2/1
  In Bus Element2/1 -> Mux/1
  In Bus Element6/1 -> Mux/2
  In Bus Element4/1 -> Mux/3
  Mux/1 -> "Incidence, Sideslip, & Airspeed"/1
  "Incidence, Sideslip, & Airspeed"/3 -> Divide/1
  In Bus Element/1 -> Divide/2
  "Incidence, Sideslip, & Airspeed"/2 -> Terminator/1
  Subsystem Reference/3 -> kss/1
  Divide/1 -> Subsystem Reference/1
  Constant1/1 -> Subsystem Reference/2
  In Bus Element5/1 -> Subsystem Reference/4
  Clock/1 -> Subsystem Reference/3

== system flat_earth_6dof/Roll Autopilot/Roll autopilot ==
  In Bus Element1 : Inport  PortName=States  Element=p
  pc : Inport  Port=2
  k1 : Inport  Port=3
  k2 : Inport  Port=4
  kss : Inport  Port=5
  Integrator : Integrator
  Product : Product
  Product1 : Product
  Product3 : Product
  Saturation : Saturate  UpperLimit=15*(pi/180)  LowerLimit=-15*(pi/180)
  Scope : Scope
  Sum2 : Sum  Inputs=|+-
  Sum3 : Sum  Inputs=|+-
  delta a : Outport
  wires:
  pc/1 -> Product/1
  Sum3/1 -> Saturation/1
  Product/1 -> Sum2/1
  In Bus Element1/1 -> Product1/2, Scope/1, Product3/1
  Sum2/1 -> Integrator/1
  Integrator/1 -> Sum3/1
  Product3/1 -> Sum3/2
  k2/1 -> Product3/2
  Saturation/1 -> delta a/1
  kss/1 -> Product/2
  Product1/1 -> Sum2/2
  k1/1 -> Product1/1

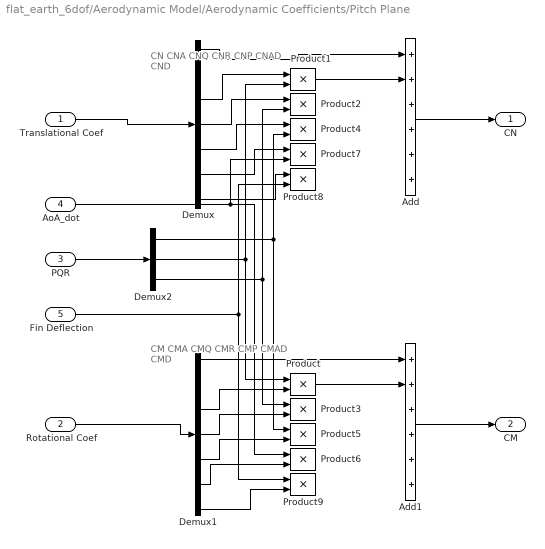
== system flat_earth_6dof/Aerodynamic Model/Aerodynamic Coefficients/Pitch Plane ==
  note: CN
      |
      | CNA
      |
      | CNQ
      |
      | CNR
      |
      | CNP
      |
      | CNAD
      |
      | CND
  note: CM
      |
      | CMA
      |
      | CMQ
      |
      | CMR
      |
      | CMP
      |
      | CMAD
      |
      | CMD
  Translational Coef : Inport
  Rotational Coef : Inport  Port=2
  PQR : Inport  Port=3
  AoA_dot : Inport  Port=4
  Fin Deflection : Inport  Port=5
  Add : Sum  Inputs=++++++
  Add1 : Sum  Inputs=++++++
  Demux : Demux  Outputs=7
  Demux1 : Demux  Outputs=7
  Demux2 : Demux  Outputs=3
  Product{,1..9} (10 alike) : Product
  CN : Outport
  CM : Outport  Port=2
  wires:
  Translational Coef/1 -> Demux/1
  Demux/1 -> Add/1
  Demux1/1 -> Add1/1
  PQR/1 -> Demux2/1
  Demux2/2 -> Product1/2, Product/1
  Product1/1 -> Add/2
  Add/1 -> CN/1
  Add1/1 -> CM/1
  Product/1 -> Add1/2
  Demux2/3 -> Product3/1, Product2/2
  Demux2/1 -> Product5/1, Product4/2
  AoA_dot/1 -> Product6/1, Product7/2
  Fin Deflection/1 -> Product9/1, Product8/2
  Rotational Coef/1 -> Demux1/1
  Demux/3 -> Product1/1
  Demux/4 -> Product2/1
  Demux/5 -> Product4/1
  Demux/6 -> Product7/1
  Demux/7 -> Product8/1
  Demux1/3 -> Product/2
  Demux1/4 -> Product3/2
  Demux1/5 -> Product5/2
  Demux1/6 -> Product6/2
  Demux1/7 -> Product9/2

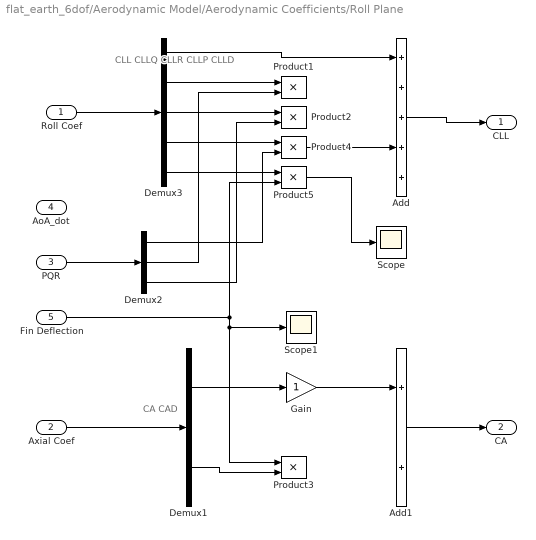
== system flat_earth_6dof/Aerodynamic Model/Aerodynamic Coefficients/Roll Plane ==
  note: CLL
      |
      | CLLQ
      |
      | CLLR
      |
      | CLLP
      |
      | CLLD
  note: CA
      |
      |
      | CAD
  Roll Coef : Inport
  Axial Coef : Inport  Port=2
  PQR : Inport  Port=3
  AoA_dot : Inport  Port=4
  Fin Deflection : Inport  Port=5
  Add : Sum  Inputs=+++++
  Add1 : Sum
  Demux1 : Demux  Outputs=2
  Demux2 : Demux  Outputs=3
  Demux3 : Demux  Outputs=5
  Gain : Gain
  Product{1..5} (5 alike) : Product
  Scope : Scope
  Scope1 : Scope
  CLL : Outport
  CA : Outport  Port=2
  wires:
  Roll Coef/1 -> Demux3/1
  PQR/1 -> Demux2/1
  Add/1 -> CLL/1
  Add1/1 -> CA/1
  Fin Deflection/1 -> Scope1/1, Product3/1, Product5/2
  Axial Coef/1 -> Demux1/1
  Demux1/1 -> Gain/1
  Demux1/2 -> Product3/2
  Demux3/2 -> Product1/1
  Demux3/3 -> Product2/1
  Demux3/4 -> Product4/1
  Demux3/5 -> Product5/1
  Demux2/2 -> Product1/2
  Demux2/3 -> Product2/2
  Demux2/1 -> Product4/2
  Product4/1 -> Add/4
  Product5/1 -> Scope/1
  Demux3/1 -> Add/1
  Gain/1 -> Add1/1

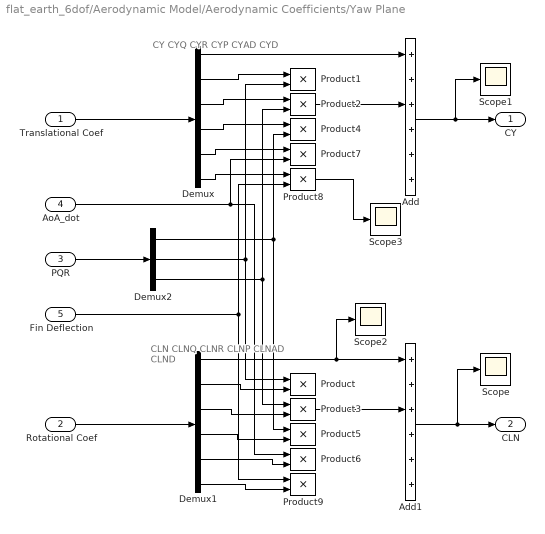
== system flat_earth_6dof/Aerodynamic Model/Aerodynamic Coefficients/Yaw Plane ==
  note: CY
      |
      | CYQ
      |
      | CYR
      |
      | CYP
      |
      | CYAD
      |
      | CYD
  note: CLN
      |
      | CLNQ
      |
      | CLNR
      |
      | CLNP
      |
      | CLNAD
      |
      | CLND
  Translational Coef : Inport
  Rotational Coef : Inport  Port=2
  PQR : Inport  Port=3
  AoA_dot : Inport  Port=4
  Fin Deflection : Inport  Port=5
  Add : Sum  Inputs=++++++
  Add1 : Sum  Inputs=++++++
  Demux : Demux  Outputs=6
  Demux1 : Demux  Outputs=6
  Demux2 : Demux  Outputs=3
  Product{,1..9} (10 alike) : Product
  Scope{,1..3} (4 alike) : Scope
  CY : Outport
  CLN : Outport  Port=2
  wires:
  Translational Coef/1 -> Demux/1
  Demux/1 -> Add/1
  Demux1/1 -> Scope2/1, Add1/1
  Demux1/2 -> Product/2
  PQR/1 -> Demux2/1
  Demux2/2 -> Product1/2, Product/1
  Demux/2 -> Product1/1
  Add/1 -> Scope1/1, CY/1
  Add1/1 -> Scope/1, CLN/1
  Demux1/3 -> Product3/2
  Demux/3 -> Product2/1
  Demux2/1 -> Product5/1, Product4/2
  Demux/4 -> Product4/1
  Demux1/4 -> Product5/2
  Product2/1 -> Add/3
  AoA_dot/1 -> Product6/1, Product7/2
  Demux1/5 -> Product6/2
  Demux/5 -> Product7/1
  Demux/6 -> Product8/1
  Fin Deflection/1 -> Product9/1, Product8/2
  Demux1/6 -> Product9/2
  Product3/1 -> Add1/3
  Rotational Coef/1 -> Demux1/1
  Product8/1 -> Scope3/1
  Demux2/3 -> Product3/1, Product2/2

== matlab function flat_earth_6dof/Intertia and Mass assignment/MATLAB Function1 ==
  data: u input; y output
function y = fcn(u)
time = u(1);
tburn = u(2);
mi = u(3);
mf = u(4);
mdot = u(5);
mass = mf;
if time < tburn
    mass = mi + mdot*time;
end
y = mass;

== matlab function flat_earth_6dof/MATLAB Function ==
  data: u input; y output
function y = fcn(u)
stop = 0;
if (u < 0)
    stop = 1;
end
y = stop;

== matlab function flat_earth_6dof/6DOF EOM/Gravity Calculation ==
  data: u input; y output
function y = fcn(u)

Re = 6357000;
g0 = 9.8;
g = g0*(Re/(Re+u))^2;

y = g;

== matlab function flat_earth_6dof/Intertia and Mass assignment/MATLAB Function2 ==
  data: u input; y output
function y = fcn(u)
on = 1;
time = u(1);
tburn = u(2);
if time > tburn
    on = 0;
end
y = on;

== matlab function flat_earth_6dof/Intertia and Mass assignment/MATLAB Function3 ==
  data: u input; y output
function y = fcn(u)
time = u(1);
tburn = u(2);
cgi = u(6);
cgf = u(7);
cgrate = (cgf - cgi)/tburn;
cg = cgf;
if time < tburn
    cg = cgi + cgrate*time;
end
y = cg;
